simulink model "if_else"  (R2021a)
settings: Solver=VariableStepAuto  StartTime=0.0  StopTime=inf  MaxStep=0.01  RelTol=1e-3
libraries: simulink x1
settings Model: Creator=Aula  LastModifiedBy=Aula

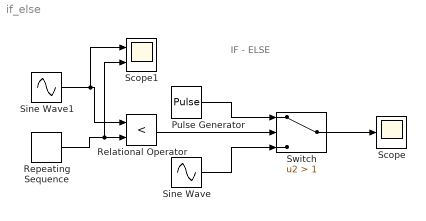
== system if_else ==
  note: IF - ELSE
  Pulse Generator : DiscretePulseGenerator  PulseType=Time based  Amplitude=5  Period=5  PulseWidth=50
  Relational Operator : RelationalOperator  Operator=<  OutDataTypeStr=boolean  RndMeth=Simplest
  Repeating Sequence : simulink/Sources/Repeating Sequence  rep_seq_t=[0 2]  rep_seq_y=[0 2]
  Scope : Scope
  Scope1 : Scope  NumInputPorts=2
  Sine Wave : Sin  Bias=2.5  Frequency=5  SampleTime=0
  Sine Wave1 : Sin  Frequency=5  SampleTime=0
  Switch : Switch  Criteria=u2 > Threshold  Threshold=1
  wires:
  Pulse Generator/1 -> Switch/1
  Sine Wave/1 -> Switch/3
  Switch/1 -> Scope/1
  Relational Operator/1 -> Switch/2
  Repeating Sequence/1 -> Scope1/2, Relational Operator/2
  Sine Wave1/1 -> Scope1/1, Relational Operator/1
